simulink model "MoreExperimentsWithGenerativeArmModelWithRestoring"  (R2013b)
settings: Solver=ode3  StartTime=0.0  StopTime=10.0  FixedStep=0.001  RelTol=1e-3
InitFcn:
  | x = -4000:1:4000;
  | startP = -0.2623;
  | endP = 0;
  | 
  | mass = 0.037;
  | A = -(startP-endP)/2; B = (endP + startP)/2;
  | 
  | y = -A + (2*A)./(1 + exp(-0.01*x)) + B;
  | 
  | fs= 1000;
  | totalTime = 8;
  | xx = 0:(1/fs):totalTime;
  | offset = 1000;
  | yMod = [-0.2623*ones(offset,1)' y(1:length(y) - offset)];
  | 
  | restoreProfile.time = xx;
  | restoreProfile.signals.values = yMod';
  | restoreProfile.signals.dimensions = 1;
StopFcn:
  | position = posProfile.signals.values;
  | velocity = velProfile.signals.values;
  | diffPosition = diff(position);
  | diffPosition(diffPosition == 0) = [];
  | 
  | 
  | position(length(diffPosition): end)= []; %remove trailing zeros. neede for midi sound.
  | velocity(length(diffPosition): end) = [];
  | 
  | position = position'; velocity = velocity';
  | position(position ~= -0.2623) = 0;
  | position(position ~= 0) = 1;
  | 
  | num = 1:length(position);
  | posVel = [num; position; velocity];
  | fid = fopen('posVel.txt','w');
  | fprintf(fid, '%5d, %6.4f %6.4f;\n', posVel);
  | fclose(fid);
  | 
  | velocityMax = velocity(min(find(position == 1)));
  | velocityMin = velocity(max(find(position == 1)));
  | 
  | fid = fopen('minMax.txt', 'w');
  | fprintf(fid, '%1d, %6.4f %6.4f;\n', 1, velocityMin, velocityMax);
  | fclose(fid);
  | 
  | robotPosition = scaledPositionProfile.signals.values;
  | save robotPosition.mat robotPosition
undefined symbols (not defined in the file or in its folder): sigbuilder_block
libraries: simulink x2
settings Model: Creator=Deepak  LastModifiedBy=Deepak

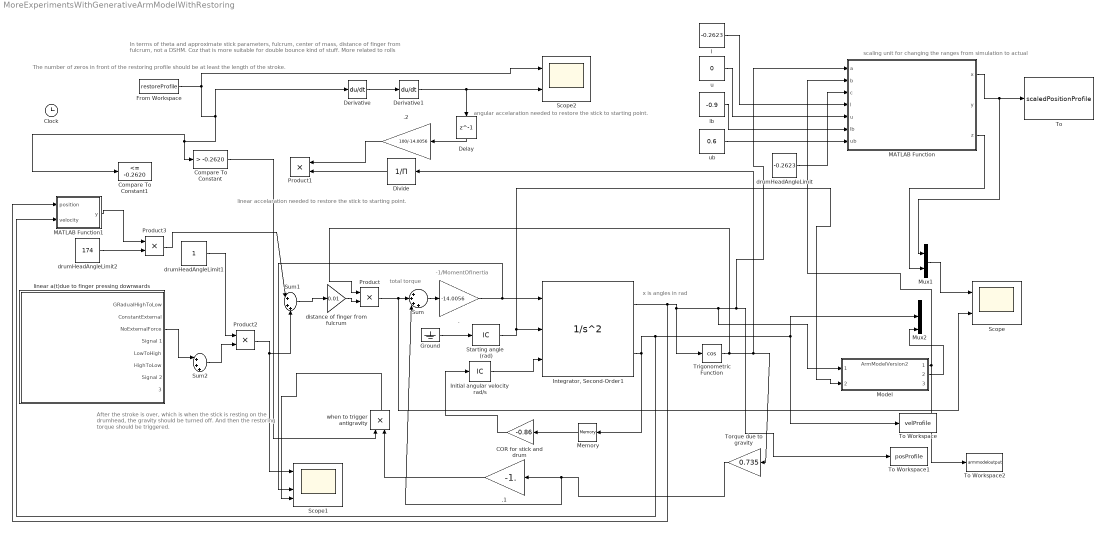
== system MoreExperimentsWithGenerativeArmModelWithRestoring ==
  note: scaling unit for changing the ranges from simulation to actual
  note: The number of zeros in front of the restoring profile should be at least the length of the stroke.
  note: angular accelaration needed to restore the stick to starting point.
  note: After the stroke is over, which is when the stick is resting on the
      | drumhead, the gravity should be turned off. And then the
      | restoring torque should be triggered.
  note: total torque
  note: -1/MomentOfInertia
  note: x is angles in rad
  note: In terms of theta and approximate stick parameters, fulcrum, center of mass, distance of finger from fulcrum, not a DSHM. Coz that is more suitable for double bounce kind of stuff. More related to rolls
  note: linear accelaration needed to restore the stick to starting point.
  . : Gain  Gain=-14.0056
  .1 : Gain  Gain=-1.
  .2 : Gain  Gain=100/-14.0056
  "COR for stick and drum " : Gain  Gain=-0.86
  Clock : Clock
  Compare To Constant : simulink/Logic and Bit Operations/Compare To Constant  relop=>  const=-0.2620  OutDataTypeStr=boolean
  Compare To Constant1 : simulink/Logic and Bit Operations/Compare To Constant  relop=<=  const=-0.2620  OutDataTypeStr=uint8
  Delay : Delay  DelayLength=1  InitialCondition=0
  Derivative : Derivative
  Derivative1 : Derivative
  Divide : Product  Inputs=/
  From Workspace : FromWorkspace  VariableName=restoreProfile  SampleTime=0
  Ground : Ground
  "Initial angular velocity rad/s " : InitialCondition  Value=0
  "Integrator, Second-Order1" : SecondOrderIntegrator  ICSourceX=external  LimitX=on  LowerLimitX=-0.2623  ICSourceDXDT=external  ReinitDXDTwhenXreachesSaturation=on
  MATLAB Function : MATLAB Function  TreatAsAtomicUnit=on
  MATLAB Function1 : MATLAB Function  TreatAsAtomicUnit=on
  Memory : Memory
  Model : ModelReference  ModelNameDialog=ArmModelVersion2.slx  SimulationMode=Normal  ModelReferenceVersion=1.94  CopyOfModelName=ArmModelVersion2.slx  DefaultDataLogging=on
  Mux1 : Mux  Inputs=2
  Mux2 : Mux  Inputs=3
  Product{,1..3} (4 alike) : Product
  Scope : Scope  NumInputPorts=2
      settings: TimeRange=10  YMin=-0.9~-1  YMax=0.09999999999999998~1  SaveName=PlotData  MaxDataPoints=50000
  Scope1 : Scope  NumInputPorts=4
      settings: TimeRange=10  YMin=-1.8~-5~-5~-5  YMax=0~5~5~5  MaxDataPoints=50000
  Scope2 : Scope  NumInputPorts=2
      settings: TimeRange=10  YMin=-1.8~-5  YMax=0~5  MaxDataPoints=60000
  Starting angle  (rad) : InitialCondition  Value=0
  Sum : Sum  Inputs=|++++
  Sum1 : Sum  Inputs=|+++
  Sum2 : Sum  Inputs=|+++
  "To " : ToWorkspace  VariableName=scaledPositionProfile  SampleTime=-1  SaveFormat=Structure
  To Workspace : ToWorkspace  VariableName=velProfile  SampleTime=-1  SaveFormat=Structure
  To Workspace1 : ToWorkspace  VariableName=posProfile  SampleTime=-1  SaveFormat=Structure
  To Workspace2 : ToWorkspace  VariableName=armmodeloutput  SampleTime=-1  SaveFormat=Structure
  Torque due to gravity : Gain  Gain=0.735
  Trigonometric Function : Trigonometry  Operator=cos
  distance of finger from fulcrum : Gain  Gain=0.01
  drumHeadAngleLimit : Constant  Value=-0.2623
  drumHeadAngleLimit1 : Constant
  drumHeadAngleLimit2 : Constant  Value=174
  l : Constant  Value=-0.2623
  lb : Constant  Value=-0.9
  linear a(t)due to finger pressing downwards : Subsystem  Tag=STV Subsys  LoadFcn=sigbuilder_block('load');  StartFcn=sigbuilder_block('start');  StopFcn=sigbuilder_block('stop');  ClipboardFcn=sigbuilder_block('clipboard');  mask(Sigbuilder block){}
      mask help: Simulink:masks:SigbuilderBlock_MD
      mask init:
      | if ~strcmp(get_param(bdroot(gcbh),'SimulationStatus'),'stopped') tuvar = sigbuilder_block('maskInit'); end
      settings: CopyFcn=sigbuilder_block('copy');  DeleteFcn=sigbuilder_block('delete');  ModelCloseFcn=sigbuilder_block('modelClose');  PreSaveFcn=sigbuilder_block('preSave');  PauseFcn=sigbuilder_block('pause');  ContinueFcn=sigbuilder_block('continue');  NameChangeFcn=sigbuilder_block('namechange');  OpenFcn=sigbuilder_block('open',[591.534 55.9559 1325.96 874.311 ]);  CloseFcn=sigbuilder_block('close');
      mask Display: plot(0, 0, 100, 100,[2, 2, 32, 32, 2], [68, 8, 8, 68, 68],[32, 2], [38, 38], [32, 19, 2],[53, 60, 44], [32, 17, 17, 2],[16, 16, 31, 31]);txt = getActiveGroup(gcbh);text(2, 100, txt,'verticalAlignment', 'top');
  "u " : Constant  Value=0
  "ub " : Constant  Value=0.6
  "when to trigger antigravity " : Product
  wires:
  "Integrator, Second-Order1"/1 -> MATLAB Function1/1(position), Model/1, MATLAB Function/1(a), To Workspace1/1, Trigonometric Function/1
  Trigonometric Function/1 -> Divide/1, Torque due to gravity/1, Product/1
  Sum/1 -> ./1
  Torque due to gravity/1 -> Sum/3, .1/1
  Ground/1 -> Starting angle  (rad)/1
  Starting angle  (rad)/1 -> Model/2, "Integrator, Second-Order1"/2
  "Initial angular velocity rad/s "/1 -> "Integrator, Second-Order1"/3
  "Integrator, Second-Order1"/2 -> Memory/1, MATLAB Function1/2(velocity), To Workspace/1, Mux2/2
  Memory/1 -> "COR for stick and drum "/1
  "COR for stick and drum "/1 -> "Initial angular velocity rad/s "/1
  Mux1/1 -> Scope/1
  distance of finger from fulcrum/1 -> Product/2
  Sum1/1 -> distance of finger from fulcrum/1
  Model/1 -> MATLAB Function/2(b), To Workspace2/1
  Model/2 -> Mux2/3
  Product/1 -> Sum/2, Scope/2
  Derivative/1 -> Derivative1/1
  From Workspace/1 -> Compare To Constant/1, Compare To Constant1/1, Derivative/1, Scope2/1
  Derivative1/1 -> Delay/1, Scope2/2
  Compare To Constant/1 -> "when to trigger antigravity "/1
  .1/1 -> "when to trigger antigravity "/2
  ./1 -> Scope1/3, "Integrator, Second-Order1"/1
  Delay/1 -> .2/1
  "when to trigger antigravity "/1 -> Scope1/4
  .2/1 -> Product1/1
  Divide/1 -> Product1/2
  drumHeadAngleLimit/1 -> MATLAB Function/3(c)
  Product2/1 -> Sum1/3, Scope1/1
  l/1 -> MATLAB Function/4(l)
  "u "/1 -> MATLAB Function/5(u)
  lb/1 -> MATLAB Function/6(lb)
  "ub "/1 -> MATLAB Function/7(ub)
  MATLAB Function/1(x) -> Mux1/1, "To "/1
  Sum2/1 -> Product2/2
  drumHeadAngleLimit1/1 -> Product2/1
  MATLAB Function/3(z) -> Mux1/2
  MATLAB Function1/1(y) -> Product3/1
  drumHeadAngleLimit2/1 -> Product3/2
  linear a(t)due to finger pressing downwards/3(NoExternalForce) -> Sum2/1
  Product3/1 -> Sum1/1

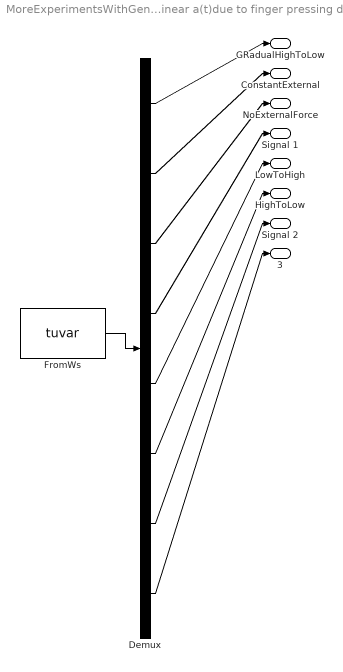
== system MoreExperimentsWithGenerativeArmModelWithRestoring/linear a(t)due to finger pressing downwards ==
  Demux : Demux  Tag=STV Demux  Outputs=8
  FromWs : FromWorkspace  Tag=STV FromWs  VariableName=tuvar  SampleTime=0
      SigBuilderData=|
      | common.afterFinalStr = 'Extrapolate'
      | common.sampleTime = 0
      | dataSet.timeRange = [0 10]
      | dataSet.name = 'Group 1'
      | sbobj.Groups.Name = 'Group 1'
      | sbobj.Groups.Signals(1).Name = 'GRadualHighToLow'
      | sbobj.Groups.Signals(1).XData = [0 10]
      | sbobj.Groups.Signals(1).YData = [520 -110]
      | sbobj.Groups.Signals(2).Name = 'ConstantExternal'
      | sbobj.Groups.Signals(2).XData = [0 10]
      | sbobj.Groups.Signals(2).YData = [101 101]
      | sbobj.Groups.Signals(3).Name = 'NoExternalForce'
      | sbobj.Groups.Signals(3).XData = [0 10]
      | sbobj.Groups.Signals(3).YData = [0 0]
      | sbobj.Groups.Signals(4).Name = 'Signal 1'
      | sbobj.Groups.Signals(4).XData = [0 0.6 0.6 0.62 0.62 10]
      | sbobj.Groups.Signals(4).YData = [0 0 200 200 0 0]
      | sbobj.Groups.Signals(5).Name = 'LowToHigh'
      | sbobj.Groups.Signals(5).XData = [0 0.6 1.3 6 6 10]
      | sbobj.Groups.Signals(5).YData = [0 0 200 1 110 0]
      | sbobj.Groups.Signals(6).Name = 'HighToLow'
      | sbobj.Groups.Signals(6).XData = [0 0.4 0.7 0.7 0.9 6 6 10]
      | sbobj.Groups.Signals(6).YData = [250 250 220 80 0 1 0 0]
      | sbobj.Groups.Signals(7).Name = 'Signal 2'
      | sbobj.Groups.Signals(7).XData = [0 0.5 1 6 6 10]
      | sbobj.Groups.Signals(7).YData = [500 500 120 -10 0 0]
      | sbobj.Groups.Signals(8).Name = '3'
      | sbobj.Groups.Signals(8).XData = [0 0.3 0.46 0.56 6 10]
      | sbobj.Groups.Signals(8).YData = [0 100 100 0 -2 0]
  GRadualHighToLow : Outport  Tag=STV Outport
  ConstantExternal : Outport  Tag=STV Outport  Port=2
  NoExternalForce : Outport  Tag=STV Outport  Port=3
  Signal 1 : Outport  Tag=STV Outport  Port=4
  LowToHigh : Outport  Tag=STV Outport  Port=5
  HighToLow : Outport  Tag=STV Outport  Port=6
  Signal 2 : Outport  Tag=STV Outport  Port=7
  3 : Outport  Tag=STV Outport  Port=8
  wires:
  FromWs/1 -> Demux/1
  Demux/1 -> GRadualHighToLow/1
  Demux/2 -> ConstantExternal/1
  Demux/3 -> NoExternalForce/1
  Demux/4 -> Signal 1/1
  Demux/5 -> LowToHigh/1
  Demux/6 -> HighToLow/1
  Demux/7 -> Signal 2/1
  Demux/8 -> 3/1

== matlab function MoreExperimentsWithGenerativeArmModelWithRestoring/MATLAB Function1 ==
  data: position input; y output; velocity input
function y = fcn(position, velocity)
%#codegen
 if(position >= -0.22 && position <= -0.2)
    if(velocity < 0)
        y = rand;
    else 
        y = 0;
    end
 else
    y = 0;    
 end
 
end

== matlab function MoreExperimentsWithGenerativeArmModelWithRestoring/MATLAB Function ==
  data: a input; b input; c input; l input; x output; u input; y output; lb input; ub input; z output
function [x,y,z] = fcn(a,b,c,l, u, lb, ub)
%#codegen

x = (ub*(a - l) + lb*(u-a))/(u-l);
y = (ub*(b - l) + lb*(u-b))/(u-l);
z = (ub*(c - l) + lb*(u-c))/(u-l);
end
